simulink model "DC_motor_client"  (R2023a)
settings: Solver=ode1  StartTime=0.0  StopTime=inf  FixedStep=0.02  RelTol=1e-3  EnableMultiTasking=on
values from neighbouring files (symbols this model uses):
  Npred = 20    [MPC_CasADi_2.m]
  Ts = 0.02    [MPC_CasADi_2.m]
libraries: simulink x10, quarc_library x10, dspbuff3 x2
settings Model: ExtModeTrigDuration=10000  Creator=marinst  LastModifiedBy=marinst
settings SolverCC: AlgebraicLoopSolver=TrustRegion  PositivePriorityOrder=on
settings DataIOCC: ReturnWorkspaceOutputs=off
settings DebuggingCC: UnconnectedInputMsg=warning  UnconnectedOutputMsg=warning  UnconnectedLineMsg=warning  ArithmeticOperatorsInVariantConditions=warning
settings ModelReferenceCC: EnableRefExpFcnMdlSchedulingChecks=on
settings SFSimCC: SimUseLocalCustomCode=off  CustomCodeUndefinedFunction=UseInterfaceOnly
settings RTWCC: RTWUseLocalCustomCode=off  Toolchain=QUARC win64 | nmake (64-bit Windows)  BuildConfiguration=Faster Runs
settings CodeAppCC: StateflowObjectComments=on
settings ConfigComp: CovMetricSettings=dswe

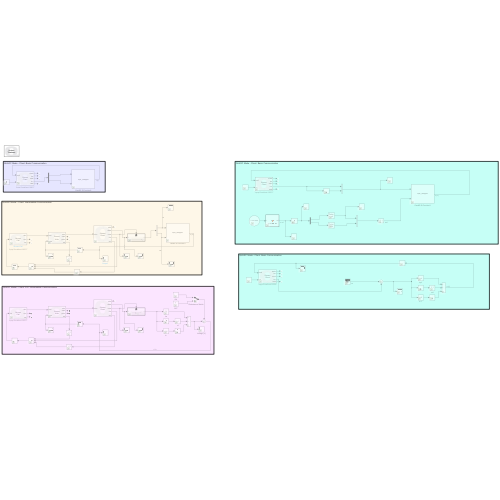
[thumbnail: Simulink's stored preview of the top-level diagram]
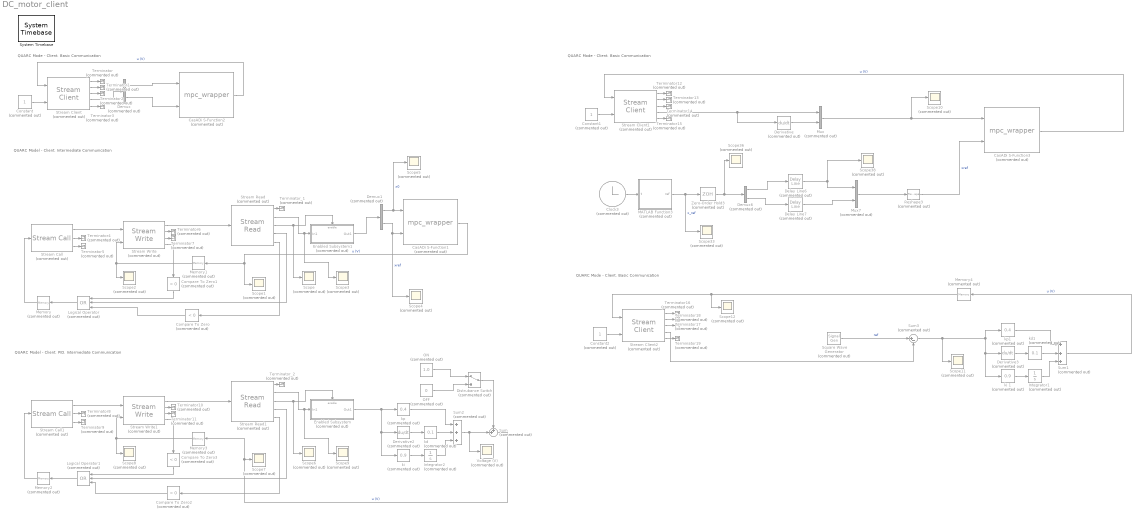
== system DC_motor_client ==
  note: QUARC Model - Client. PID. Intermediate Communication
  note: QUARC Model - Client. Intermediate Communication
  note: QUARC Mode - Client. Basic Communication
  note: QUARC Mode - Client. Basic Communication
  note: QUARC Mode - Client. Basic Communication
  CasADi S-Function1 : S-Function  Commented=on  FunctionName=mpc_wrapper  SFunctionDeploymentMode=off  EnableBusSupport=off
  CasADi S-Function2 : S-Function  Commented=on  FunctionName=mpc_wrapper  SFunctionDeploymentMode=off  EnableBusSupport=off
  CasADi S-Function3 : S-Function  Commented=on  FunctionName=mpc_wrapper  SFunctionDeploymentMode=off  EnableBusSupport=off
  Clock3 : Clock  Commented=on
  Compare To Zero{,1..3} (4 alike) : simulink/Logic and Bit Operations/Compare To Zero  Commented=on  relop=<  OutDataTypeStr=boolean
  Constant : Constant  Commented=on
  Constant1 : Constant  Commented=on
  Constant2 : Constant  Commented=on
  Delay Line6 : dspbuff3/Delay Line  Commented=on  siz=Npred+1  ic=0  directfeed=off  enable_output=off  hold_output=off  OutputFrames=off
  Delay Line7 : dspbuff3/Delay Line  Commented=on  siz=Npred+1  ic=0  directfeed=off  enable_output=off  hold_output=off  OutputFrames=off
  Demux : Demux  Commented=on  Outputs=[2 42]
  Demux1 : Demux  Commented=on  Outputs=[2 42]
  Demux6 : Demux  Commented=on  Outputs=2
  Derivative : Derivative  Commented=on
  Derivative2 : Derivative  Commented=on
  Derivative3 : Derivative  Commented=on
  Distrubance Switch : ManualSwitch  Commented=on
  Enabled Subsystem : Subsystem  Commented=on  TreatAsAtomicUnit=on
  Enabled Subsystem1 : Subsystem  Commented=on  TreatAsAtomicUnit=on
  Integrator1 : Integrator  Commented=on
  Integrator2 : Integrator  Commented=on
  Logical Operator : Logic  Commented=on  Operator=OR  Inputs=3  AllPortsSameDT=off  OutDataTypeStr=boolean
  Logical Operator1 : Logic  Commented=on  Operator=OR  Inputs=3  AllPortsSameDT=off  OutDataTypeStr=boolean
  MATLAB Function3 : MATLAB Function  Commented=on  TreatAsAtomicUnit=on
  Memory{,1..4} (5 alike) : Memory  Commented=on
  Mux : Mux  Commented=on  Inputs=2
  Mux7 : Mux  Commented=on  Inputs=2
  OFF : Constant  Commented=on  Value=0
  ON : Constant  Commented=on  Value=1.0
  Reshape3 : Reshape  Commented=on
  Scope{,1..12,33,36,38} (16 alike) : Scope  Commented=on
  Square Wave Generator : SignalGenerator  Commented=on  WaveForm=square  Amplitude=pi/4  Frequency=0.5
  Stream Call : quarc_library/Communications/Intermediate/Stream Call  Commented=on  uri_source=Specify via dialog (do not evaluate)  uri=tcpip://localhost:18001  send_buffer_size=8000  receive_buffer_size=8000  byte_order=little endian (Intel - LSB first)  sample_time=qc_get_step_size  non_blocking=on  active=on
      settings: AttributesFormatString="\"tcpip://localhost:18001\""  SourceProductName=QUARC Targets
  Stream Call1 : quarc_library/Communications/Intermediate/Stream Call  Commented=on  uri_source=Specify via dialog (do not evaluate)  uri=tcpip://localhost:18001  send_buffer_size=8000  receive_buffer_size=8000  byte_order=little endian (Intel - LSB first)  sample_time=qc_get_step_size  non_blocking=on  active=on
      settings: AttributesFormatString="\"tcpip://localhost:18001\""  SourceProductName=QUARC Targets
  Stream Client : quarc_library/Communications/Basic/Stream Client  Commented=on  uri_source=Specify via dialog (do not evaluate)  uri=tcpip://localhost:18001  send_buffer_size=1460  receive_buffer_size=1460  byte_order=little endian (Intel - LSB first)  optimization=Minimum latency  send_options=Send most recent data  receive_options=Receive all data  default_value=[0]  sample_time=qc_get_step_size  active=off  implementation=Use blocking I/O in a separate thread  send_fifo_size=1000  receive_fifo_size=1000  send_priority=0  receive_priority=0  send_dimensions=off  receive_dimensions=off  max_dimensions=-1  data_type=Inherited via back propagation  type_expr=BusObject
      settings: AttributesFormatString="\"tcpip://localhost:18001\""
  Stream Client1 : quarc_library/Communications/Basic/Stream Client  Commented=on  uri_source=Specify via dialog (do not evaluate)  uri=tcpip://localhost:18001  send_buffer_size=1460  receive_buffer_size=1460  byte_order=little endian (Intel - LSB first)  optimization=Minimum latency  send_options=Send most recent data  receive_options=Receive all data  default_value=[0]  sample_time=qc_get_step_size  active=off  implementation=Use blocking I/O in a separate thread  send_fifo_size=1000  receive_fifo_size=1000  send_priority=0  receive_priority=0  send_dimensions=off  receive_dimensions=off  max_dimensions=-1  data_type=Inherited via back propagation  type_expr=BusObject
      settings: AttributesFormatString="\"tcpip://localhost:18001\""
  Stream Client2 : quarc_library/Communications/Basic/Stream Client  Commented=on  uri_source=Specify via dialog (do not evaluate)  uri=tcpip://localhost:18002  send_buffer_size=1460  receive_buffer_size=1460  byte_order=little endian (Intel - LSB first)  optimization=Minimum latency  send_options=Send most recent data  receive_options=Receive most recent data  default_value=[0]  sample_time=qc_get_step_size  active=off  implementation=Use blocking I/O in a separate thread  send_fifo_size=1000  receive_fifo_size=1000  send_priority=0  receive_priority=0  send_dimensions=off  receive_dimensions=off  max_dimensions=-1  data_type=Inherited via back propagation  type_expr=BusObject
      settings: AttributesFormatString="\"tcpip://localhost:18002\""
  Stream Read : quarc_library/Communications/Intermediate/Stream Read  Commented=on  data_type=double  type_expr=BusObject  num_elements=[1 44]  receive_dims=off
      settings: SourceProductName=QUARC Targets
  Stream Read1 : quarc_library/Communications/Intermediate/Stream Read  Commented=on  data_type=double  type_expr=BusObject  num_elements=1  receive_dims=off
      settings: SourceProductName=QUARC Targets
  Stream Write : quarc_library/Communications/Intermediate/Stream Write  Commented=on  optimization=Minimizing latency  send_dims=off
      settings: SourceProductName=QUARC Targets
  Stream Write1 : quarc_library/Communications/Intermediate/Stream Write  Commented=on  optimization=Minimizing latency  send_dims=off
      settings: SourceProductName=QUARC Targets
  Sum : Sum  Commented=on  Inputs=++|
  Sum1 : Sum  Commented=on  Inputs=+++
  Sum2 : Sum  Commented=on  Inputs=+++
  Sum3 : Sum  Commented=on  Inputs=|+-
  System Timebase : quarc_library/Advanced/Timing/System Timebase  stop_on_overrun=off
      settings: SourceProductName=QUARC Targets
  Terminator{,1..19} (20 alike) : Terminator  Commented=on
  Terminator_1 : Terminator  Commented=on
  Terminator_2 : Terminator  Commented=on
  Voltage (V) : Scope  Commented=on
  Zero-Order Hold3 : ZeroOrderHold  Commented=on  SampleTime=Ts
  kd : simulink/Math Operations/Slider Gain  Commented=on  gain=0.1  low=-1  high=500
  kd1 : simulink/Math Operations/Slider Gain  Commented=on  gain=0.1  low=-1  high=500
  "ki " : simulink/Math Operations/Slider Gain  Commented=on  gain=0.9  low=0  high=500
  ki 1 : simulink/Math Operations/Slider Gain  Commented=on  gain=0.9  low=0  high=500
  kp : simulink/Math Operations/Slider Gain  Commented=on  gain=0.4  low=0  high=500
  kp1 : simulink/Math Operations/Slider Gain  Commented=on  gain=0.4  low=0  high=500
  wires:
  Stream Client/4 -> Demux/1
  Demux/2 -> CasADi S-Function2/2
  Demux/1 -> CasADi S-Function2/1
  CasADi S-Function2/1 -> Stream Client/1  "u (V)"
  Constant/1 -> Stream Client/2
  Stream Client/1 -> Terminator/1
  Stream Client/2 -> Terminator1/1
  Stream Client/3 -> Terminator2/1
  Stream Client/5 -> Terminator3/1
  Stream Read/3 -> Enabled Subsystem1/Enable, Scope/1
  Stream Read/5 -> Compare To Zero/1
  Stream Read/1 -> Terminator_1/1
  Memory/1 -> Stream Call/1
  Stream Write/1 -> Stream Read/1
  Stream Write/4 -> Compare To Zero1/1
  Logical Operator/1 -> Memory/1
  Stream Read/4 -> Logical Operator/2
  Stream Write/3 -> Terminator7/1
  Stream Call/2 -> Terminator4/1
  Stream Call/1 -> Stream Write/1
  Stream Call/3 -> Terminator5/1
  Demux1/1 -> Scope5/1, CasADi S-Function1/1  "x0"
  Demux1/2 -> Scope4/1, CasADi S-Function1/2  "xref"
  Memory1/1 -> Scope2/1, Stream Write/2
  Stream Read/2 -> Enabled Subsystem1/1(In1), Scope3/1
  Enabled Subsystem1/1(Out1) -> Demux1/1
  Stream Write/2 -> Terminator6/1
  Compare To Zero/1 -> Logical Operator/3
  Compare To Zero1/1 -> Logical Operator/1
  CasADi S-Function1/1 -> Memory1/1, Scope1/1  "u (V)"
  Enabled Subsystem/1(Out1) -> "ki "/1, Derivative2/1, kp/1
  Distrubance Switch/1 -> Sum/1
  Sum2/1 -> Voltage (V)/1, Sum/2
  ON/1 -> Distrubance Switch/1
  Derivative2/1 -> kd/1
  OFF/1 -> Distrubance Switch/2
  "ki "/1 -> Integrator2/1
  Integrator2/1 -> Sum2/3
  kd/1 -> Sum2/2
  kp/1 -> Sum2/1
  Stream Call1/1 -> Stream Write1/1
  Compare To Zero3/1 -> Logical Operator1/1
  Stream Write1/2 -> Terminator10/1
  Compare To Zero2/1 -> Logical Operator1/3
  Stream Read1/1 -> Terminator_2/1
  Sum/1 -> Memory3/1, Scope7/1  "u (V)"
  Stream Read1/2 -> Enabled Subsystem/1(In1), Scope9/1
  Stream Read1/5 -> Compare To Zero2/1
  Stream Call1/2 -> Terminator8/1
  Memory3/1 -> Scope8/1, Stream Write1/2
  Stream Call1/3 -> Terminator9/1
  Stream Write1/1 -> Stream Read1/1
  Logical Operator1/1 -> Memory2/1
  Stream Write1/4 -> Compare To Zero3/1
  Memory2/1 -> Stream Call1/1
  Stream Read1/3 -> Enabled Subsystem/Enable, Scope6/1
  Stream Write1/3 -> Terminator11/1
  Stream Read1/4 -> Logical Operator1/2
  CasADi S-Function3/1 -> Stream Client1/1  "u (V)"
  Stream Client1/1 -> Terminator12/1
  Stream Client1/2 -> Terminator13/1
  Stream Client1/5 -> Terminator15/1
  Stream Client1/3 -> Terminator14/1
  Constant1/1 -> Stream Client1/2
  MATLAB Function3/1(ref) -> Scope33/1, Zero-Order Hold3/1  "x_ref"
  Delay Line7/1 -> Mux7/2
  Zero-Order Hold3/1 -> Demux6/1, Scope36/1
  Demux6/1 -> Delay Line6/1
  Mux7/1 -> Reshape3/1
  Demux6/2 -> Delay Line7/1
  Delay Line6/1 -> Scope38/1, Mux7/1
  Clock3/1 -> MATLAB Function3/1(t)
  Reshape3/1 -> CasADi S-Function3/2  "xref"
  Mux/1 -> Scope10/1, CasADi S-Function3/1
  Derivative/1 -> Mux/2
  Stream Client1/4 -> Derivative/1, Mux/1
  Stream Client2/3 -> Terminator18/1
  Constant2/1 -> Stream Client2/2
  Stream Client2/2 -> Terminator17/1
  Stream Client2/1 -> Terminator16/1
  Sum1/1 -> Memory4/1  "u (V)"
  Stream Client2/5 -> Terminator19/1
  ki 1/1 -> Integrator1/1
  kd1/1 -> Sum1/2
  kp1/1 -> Sum1/1
  Sum3/1 -> Scope11/1, kp1/1, ki 1/1, Derivative3/1
  Derivative3/1 -> kd1/1
  Integrator1/1 -> Sum1/3
  Square Wave Generator/1 -> Sum3/1  "ref"
  Stream Client2/4 -> Sum3/2
  Memory4/1 -> Stream Client2/1, Scope12/1

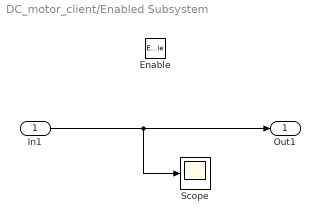
== system DC_motor_client/Enabled Subsystem ==
  In1 : Inport
  Enable : EnablePort
  Scope : Scope
  Out1 : Outport
  wires:
  In1/1 -> Scope/1, Out1/1

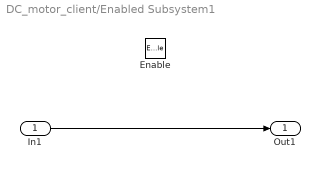
== system DC_motor_client/Enabled Subsystem1 ==
  In1 : Inport
  Enable : EnablePort
  Out1 : Outport
  wires:
  In1/1 -> Out1/1

== matlab function DC_motor_client/MATLAB Function3 ==
  data: t input; ref output
function ref = generate_ref(t)
    amp = pi/4;
    freq = 0.5;
    ref1 = -amp * square(2*pi*freq*t);
    ref2 = 0;
    ref = [ref1; ref2];
end
